simulink model "mainV02_3"  (R2016b)
settings: Solver=VariableStepAuto  StartTime=0.0  StopTime=inf  MaxStep=0.2  RelTol=1e-2
undefined symbols (not defined in the file): checks, delta_e, deltae_degrees, deltat_1, deltat_2, deltat_3, deltat_4, deltat_5, Earth, ft, initialValues, LD, m, Newton, Raphson, s, WGS84
libraries: aerolibutil x8, aerolibasang x5, aerolib6dof2 x4, aerolib6dofsys x3, aerolibtransform2 x3, aerolibbdyn x3, aerolibconvert2 x3, aerolibconvert x2, aerolibatmos2 x1, aerolibobsolete x1, aerolibadyn x1, vrlib x1
(part 2 of 3)

== system mainV02_3/LIBIS Plant/calc alpha_dot ==
  q : Inport
  alpha,beta : Inport  Port=2
  Ab : Inport  Port=3
  Vw : Inport  Port=4
  Constant : Constant  Value=0
  Direction Cosine Matrix Body to Wind : aerolibtransform2/Direction Cosine Matrix Body to Wind
  Product1 : Product  Multiplication=Matrix(*)  SaturateOnIntegerOverflow=on  InputSameDT=on  OutDataTypeStr=Inherit: Same as first input
  Product2 : Product  Inputs=*/  SaturateOnIntegerOverflow=on  InputSameDT=on  OutDataTypeStr=Inherit: Same as first input
  Selector2 : Selector  IndexMode=Zero-based  InputPortWidth=3  IndexOptions=Index vector (dialog)  Indices=2  OutputSizes=1
  Selector3 : Selector  IndexMode=Zero-based  InputPortWidth=3  IndexOptions=Index vector (dialog)  Indices=0  OutputSizes=1
  Sum : Sum  Inputs=++|
  Switch : Switch  Criteria=u2 > Threshold
  Transpose1 : Math  Operator=transpose  SaturateOnIntegerOverflow=on
  Transpose2 : Math  Operator=transpose  SaturateOnIntegerOverflow=on
  alpha_dot : Outport
  wires:
  Direction Cosine Matrix Body to Wind/1 -> Transpose1/1
  Transpose1/1 -> Product1/1
  Product1/1 -> Selector2/1
  Selector2/1 -> Product2/1
  alpha,beta/1 -> Direction Cosine Matrix Body to Wind/1
  q/1 -> Sum/1
  Sum/1 -> alpha_dot/1
  Vw/1 -> Selector3/1
  Selector3/1 -> Switch/2, Product2/2
  Product2/1 -> Switch/1
  Switch/1 -> Sum/2
  Constant/1 -> Switch/3
  Transpose2/1 -> Product1/2
  Ab/1 -> Transpose2/1

== system mainV02_3/Visualization/Airspeed Indicator ==

== system mainV02_3/Visualization/Altimeter ==

== system mainV02_3/Visualization/Artificial Horizon ==

== system mainV02_3/Visualization/Axes to VR Axes ==
  Xe : Inport
  Concatenate : Concatenate  NumInputs=3
  Demux : Demux  Outputs=3
  rad-->deg : Gain  Gain=-1  SaturateOnIntegerOverflow=on  OutDataTypeStr=Inherit: Same as input  ParamDataTypeStr=Inherit: Same as input
  rad-->deg1 : Gain  Gain=-1  SaturateOnIntegerOverflow=on  OutDataTypeStr=Inherit: Same as input  ParamDataTypeStr=Inherit: Same as input
  Xe VR : Outport
  wires:
  Xe/1 -> Demux/1
  Demux/1 -> Concatenate/1
  Demux/2 -> rad-->deg/1
  Demux/3 -> rad-->deg1/1
  Concatenate/1 -> Xe VR/1
  rad-->deg1/1 -> Concatenate/2
  rad-->deg/1 -> Concatenate/3

== system mainV02_3/Visualization/Climb Rate Indicator ==

== system mainV02_3/Visualization/Euler to VR ==
  Euler Angles : Inport
  Axis Angle Vector : Subsystem
  Demux : Demux  Outputs=3
  Mux : Mux  Inputs=2
  Mux1 : Mux  Inputs=2
  Mux2 : Mux  Inputs=2
  Quaternion Multiplication (Pitch & Yaw) : aerolibutil/Quaternion Multiplication
  Quaternion Multiplication (Roll) : aerolibutil/Quaternion Multiplication
  Quaternion Normalization : Subsystem
  Quaternion Normalization1 : Subsystem
  Quaternion Normalization2 : Subsystem
  Vr Pitch Axes : Constant  Value=[0 0 1]
  Vr Roll Axes : Constant  Value=[1 0 0]
  Vr Yaw Axes : Constant  Value=[0 -1 0]
  Axis Angle : Outport
  wires:
  Quaternion Multiplication (Roll)/1 -> Axis Angle Vector/1(e0)
  Quaternion Multiplication (Pitch & Yaw)/1 -> Quaternion Multiplication (Roll)/2
  Axis Angle Vector/1(e0_norm) -> Axis Angle/1
  Quaternion Normalization/1(e0_norm) -> Quaternion Multiplication (Roll)/1
  Quaternion Normalization2/1(e0_norm) -> Quaternion Multiplication (Pitch & Yaw)/1
  Quaternion Normalization1/1(e0_norm) -> Quaternion Multiplication (Pitch & Yaw)/2
  Mux2/1 -> Quaternion Normalization2/1(e0)
  Mux1/1 -> Quaternion Normalization1/1(e0)
  Mux/1 -> Quaternion Normalization/1(e0)
  Demux/3 -> Mux2/1
  Vr Yaw Axes/1 -> Mux2/2
  Demux/2 -> Mux1/1
  Vr Pitch Axes/1 -> Mux1/2
  Demux/1 -> Mux/1
  Vr Roll Axes/1 -> Mux/2
  Euler Angles/1 -> Demux/1

== system mainV02_3/Visualization/Heading Indicator ==

== system mainV02_3/Visualization/Subsystem ==
  "X_ned " : Inport
  Euler_angles : Inport  Port=2
  V_body : Inport  Port=3
  V_ned : Inport  Port=4
  Angle Conversion : aerolibconvert2/Angle Conversion  IU=rad  OU=deg
  Angle Conversion1 : aerolibconvert2/Angle Conversion  IU=rad  OU=deg
  Climbrate : Selector  IndexMode=Zero-based  InputPortWidth=3  IndexOptions=Index vector (dialog)  Indices=2  OutputSizes=1
  Concatenate : Concatenate
  Dot Product : DotProduct  SaturateOnIntegerOverflow=on  OutDataTypeStr=Inherit: Inherit via internal rule
  Flightpath Angle : Subsystem
  Heading : Selector  IndexMode=Zero-based  InputPortWidth=3  IndexOptions=Index vector (dialog)  Indices=2  OutputSizes=1
  Height : Selector  IndexMode=Zero-based  InputPortWidth=3  IndexOptions=Index vector (dialog)  Indices=2  OutputSizes=1
  Length Conversion : aerolibconvert2/Length Conversion  IU=m  OU=ft
  Roll Angle : Selector  IndexMode=Zero-based  InputPortWidth=3  IndexOptions=Index vector (dialog)  Indices=0  OutputSizes=1
  Velocity Conversion : aerolibconvert/Velocity Conversion  IU=m/s  OU=kts
  Velocity Conversion1 : aerolibconvert/Velocity Conversion  IU=m/s  OU=ft/s
  rad-->deg1 : Gain  Gain=-1  SaturateOnIntegerOverflow=on  OutDataTypeStr=Inherit: Same as input  ParamDataTypeStr=Inherit: Same as input
  rad-->deg2 : Gain  Gain=-1  SaturateOnIntegerOverflow=on  OutDataTypeStr=Inherit: Same as input  ParamDataTypeStr=Inherit: Same as input
  rad-->deg3 : Gain  Gain=60  SaturateOnIntegerOverflow=on  OutDataTypeStr=Inherit: Same as input  ParamDataTypeStr=Inherit: Same as input
  vt : Sqrt  SaturateOnIntegerOverflow=on
  Airspeed (kts) : Outport
  Height (ft) : Outport  Port=2
  Roll Flightpath (deg) : Outport  Port=3
  Climb Rate (ft/min) : Outport  Port=4
  Heading (deg) : Outport  Port=5
  wires:
  Velocity Conversion1/1 -> rad-->deg3/1
  rad-->deg3/1 -> Climb Rate (ft/min)/1
  V_ned/1 -> Flightpath Angle/1(Ve), Climbrate/1
  Flightpath Angle/1(gamma) -> Concatenate/2
  rad-->deg2/1 -> Velocity Conversion1/1
  Length Conversion/1 -> Height (ft)/1
  Angle Conversion1/1 -> Roll Flightpath (deg)/1
  Height/1 -> rad-->deg1/1
  Angle Conversion/1 -> Heading (deg)/1  "Heading"
  Heading/1 -> Angle Conversion/1
  Velocity Conversion/1 -> Airspeed (kts)/1
  Dot Product/1 -> vt/1
  Roll Angle/1 -> Concatenate/1
  V_body/1 -> Dot Product/2, Dot Product/1
  Concatenate/1 -> Angle Conversion1/1
  vt/1 -> Velocity Conversion/1
  Climbrate/1 -> rad-->deg2/1
  rad-->deg1/1 -> Length Conversion/1
  Euler_angles/1 -> Roll Angle/1, Heading/1
  "X_ned "/1 -> Height/1

== system mainV02_3/LIBIS Plant/Aerodynamics/CD ==
  prelook-ups : Inport
  plantData : Inport  Port=2
  actuators : Inport  Port=3
  Add : Sum  Inputs=+++++++
  Bus Selector : BusSelector  OutputSignals=alpha,alpha_dot,Omega_body.q
  Bus Selector1 : BusSelector  OutputSignals=alpha,alt,xcg,deltae,deltar,deltafr,deltafl
  Bus Selector2 : BusSelector  OutputSignals=deltae,deltafr,deltafl
  CD0 : Interpolation_n-D  NumberOfTableDimensions=7  Table=LD.Stability.CD0  RequireIndexFractionAsBus=on  InternalRulePriority=Speed
      settings: InputPortMap=u0,u1,u2,u3,u4,u5,u6
  CDalpha : Interpolation_n-D  NumberOfTableDimensions=7  Table=LD.Stability.CDalpha  RequireIndexFractionAsBus=on  InternalRulePriority=Speed
      settings: InputPortMap=u0,u1,u2,u3,u4,u5,u6
  CDalpha_dot : Interpolation_n-D  NumberOfTableDimensions=7  Table=LD.Stability.CDalpha_dot  RequireIndexFractionAsBus=on  InternalRulePriority=Speed
      settings: InputPortMap=u0,u1,u2,u3,u4,u5,u6
  CDdeltae : Interpolation_n-D  NumberOfTableDimensions=7  Table=LD.Stability.CDdeltae  RequireIndexFractionAsBus=on  InternalRulePriority=Speed
      settings: InputPortMap=u0,u1,u2,u3,u4,u5,u6
  CDdeltafl : Interpolation_n-D  NumberOfTableDimensions=7  Table=LD.Stability.CDdeltafl  RequireIndexFractionAsBus=on  InternalRulePriority=Speed
      settings: InputPortMap=u0,u1,u2,u3,u4,u5,u6
  CDdeltafr : Interpolation_n-D  NumberOfTableDimensions=7  Table=LD.Stability.CDdeltafr  RequireIndexFractionAsBus=on  InternalRulePriority=Speed
      settings: InputPortMap=u0,u1,u2,u3,u4,u5,u6
  CDq : Interpolation_n-D  NumberOfTableDimensions=7  Table=LD.Stability.CDq  RequireIndexFractionAsBus=on  InternalRulePriority=Speed
      settings: InputPortMap=u0,u1,u2,u3,u4,u5,u6
  Product{,1..5} (6 alike) : Product
  CD : Outport
  wires:
  prelook-ups/1 -> Bus Selector1/1
  CD0/1 -> Add/1
  Add/1 -> CD/1
  plantData/1 -> Bus Selector/1
  actuators/1 -> Bus Selector2/1
  CDalpha/1 -> Product/1
  Product/1 -> Add/2
  Bus Selector/1 -> Product/2  "<alpha>"
  Bus Selector2/1 -> Product3/2  "<deltae>"
  CDdeltae/1 -> Product3/1
  Product3/1 -> Add/5
  Product2/1 -> Add/4
  Product1/1 -> Add/3
  CDalpha_dot/1 -> Product1/1
  CDq/1 -> Product2/1
  Bus Selector/3 -> Product2/2  "<q>"
  Bus Selector/2 -> Product1/2  "<alpha_dot>"
  Bus Selector1/7 -> CD0/7, CDdeltafl/7, CDdeltafr/7, CDdeltae/7, CDq/7, CDalpha_dot/7, CDalpha/7  "<deltafl>"
  Bus Selector1/6 -> CD0/6, CDdeltafl/6, CDdeltafr/6, CDdeltae/6, CDq/6, CDalpha_dot/6, CDalpha/6  "<deltafr>"
  Bus Selector1/5 -> CD0/5, CDdeltafl/5, CDdeltafr/5, CDdeltae/5, CDq/5, CDalpha_dot/5, CDalpha/5  "<deltar>"
  Bus Selector1/4 -> CD0/4, CDdeltafl/4, CDdeltafr/4, CDdeltae/4, CDq/4, CDalpha_dot/4, CDalpha/4  "<deltae>"
  Bus Selector1/2 -> CD0/2, CDdeltafl/2, CDdeltafr/2, CDdeltae/2, CDq/2, CDalpha_dot/2, CDalpha/2  "<alt>"
  Bus Selector1/3 -> CD0/3, CDdeltafl/3, CDdeltafr/3, CDdeltae/3, CDq/3, CDalpha_dot/3, CDalpha/3  "<xcg>"
  Bus Selector1/1 -> CD0/1, CDdeltafl/1, CDdeltafr/1, CDdeltae/1, CDq/1, CDalpha_dot/1, CDalpha/1  "<alpha>"
  Bus Selector2/3 -> Product5/2  "<deltafl>"
  CDdeltafl/1 -> Product5/1
  Product5/1 -> Add/7
  Product4/1 -> Add/6
  CDdeltafr/1 -> Product4/1
  Bus Selector2/2 -> Product4/2  "<deltafr>"

== system mainV02_3/LIBIS Plant/Aerodynamics/CL ==
  prelook-ups : Inport
  plantData : Inport  Port=2
  actuators1 : Inport  Port=3
  Add : Sum  Inputs=+++++++
  Bus Selector : BusSelector  OutputSignals=alpha,alpha_dot,Omega_body.q
  Bus Selector1 : BusSelector  OutputSignals=alpha,alt,xcg,deltae,deltar,deltafr,deltafl
  Bus Selector3 : BusSelector  OutputSignals=deltae,deltafr,deltafl
  CL0 : Interpolation_n-D  NumberOfTableDimensions=7  Table=LD.Stability.CL0  RequireIndexFractionAsBus=on  InternalRulePriority=Speed
      settings: InputPortMap=u0,u1,u2,u3,u4,u5,u6
  CLalpha : Interpolation_n-D  NumberOfTableDimensions=7  Table=LD.Stability.CLalpha  RequireIndexFractionAsBus=on  InternalRulePriority=Speed
      settings: InputPortMap=u0,u1,u2,u3,u4,u5,u6
  CLalpha_dot : Interpolation_n-D  NumberOfTableDimensions=7  Table=LD.Stability.CLalpha_dot  RequireIndexFractionAsBus=on  InternalRulePriority=Speed
      settings: InputPortMap=u0,u1,u2,u3,u4,u5,u6
  CLdeltae : Interpolation_n-D  NumberOfTableDimensions=7  Table=LD.Stability.CLdeltae  RequireIndexFractionAsBus=on  InternalRulePriority=Speed
      settings: InputPortMap=u0,u1,u2,u3,u4,u5,u6
  CLdeltafl : Interpolation_n-D  NumberOfTableDimensions=7  Table=LD.Stability.CLdeltafl  RequireIndexFractionAsBus=on  InternalRulePriority=Speed
      settings: InputPortMap=u0,u1,u2,u3,u4,u5,u6
  CLdeltafr : Interpolation_n-D  NumberOfTableDimensions=7  Table=LD.Stability.CLdeltafr  RequireIndexFractionAsBus=on  InternalRulePriority=Speed
      settings: InputPortMap=u0,u1,u2,u3,u4,u5,u6
  CLq : Interpolation_n-D  NumberOfTableDimensions=7  Table=LD.Stability.CLq  RequireIndexFractionAsBus=on  InternalRulePriority=Speed
      settings: InputPortMap=u0,u1,u2,u3,u4,u5,u6
  Product{,1..5} (6 alike) : Product
  CL : Outport
  wires:
  prelook-ups/1 -> Bus Selector1/1
  CL0/1 -> Add/1
  Add/1 -> CL/1
  plantData/1 -> Bus Selector/1
  CLalpha/1 -> Product/1
  CLalpha_dot/1 -> Product1/1
  CLq/1 -> Product2/1
  CLdeltae/1 -> Product3/1
  Product/1 -> Add/2
  Product1/1 -> Add/3
  Product2/1 -> Add/4
  Product3/1 -> Add/5
  Bus Selector/1 -> Product/2  "<alpha>"
  Bus Selector/2 -> Product1/2  "<alpha_dot>"
  Bus Selector/3 -> Product2/2  "<q>"
  actuators1/1 -> Bus Selector3/1
  Bus Selector3/3 -> Product5/2  "<deltafl>"
  CLdeltafl/1 -> Product5/1
  Product5/1 -> Add/7
  Product4/1 -> Add/6
  CLdeltafr/1 -> Product4/1
  Bus Selector3/2 -> Product4/2  "<deltafr>"
  Bus Selector3/1 -> Product3/2  "<deltae>"
  Bus Selector1/7 -> CL0/7, CLalpha/7, CLalpha_dot/7, CLdeltafl/7, CLdeltafr/7, CLdeltae/7, CLq/7  "<deltafl>"
  Bus Selector1/6 -> CL0/6, CLalpha/6, CLalpha_dot/6, CLdeltafl/6, CLdeltafr/6, CLdeltae/6, CLq/6  "<deltafr>"
  Bus Selector1/5 -> CL0/5, CLalpha/5, CLalpha_dot/5, CLdeltafl/5, CLdeltafr/5, CLdeltae/5, CLq/5  "<deltar>"
  Bus Selector1/4 -> CL0/4, CLalpha/4, CLalpha_dot/4, CLq/4, CLdeltafl/4, CLdeltafr/4, CLdeltae/4  "<deltae>"
  Bus Selector1/2 -> CL0/2, CLalpha/2, CLalpha_dot/2, CLq/2, CLdeltafl/2, CLdeltafr/2, CLdeltae/2  "<alt>"
  Bus Selector1/3 -> CL0/3, CLalpha/3, CLalpha_dot/3, CLq/3, CLdeltafl/3, CLdeltafr/3, CLdeltae/3  "<xcg>"
  Bus Selector1/1 -> CL0/1, CLalpha/1, CLalpha_dot/1, CLq/1, CLdeltafl/1, CLdeltafr/1, CLdeltae/1  "<alpha>"

== system mainV02_3/LIBIS Plant/Aerodynamics/CY ==
  prelook-ups : Inport
  plantData : Inport  Port=2
  actuators : Inport  Port=3
  Add : Sum  Inputs=++++++
  Bus Selector : BusSelector  OutputSignals=beta,Omega_body.p,Omega_body.r
  Bus Selector1 : BusSelector  OutputSignals=alpha,alt,xcg,deltae,deltar,deltafr,deltafl
  Bus Selector2 : BusSelector  OutputSignals=deltar,deltafr,deltafl
  CYbeta : Interpolation_n-D  NumberOfTableDimensions=7  Table=LD.Stability.CYbeta  RequireIndexFractionAsBus=on  InternalRulePriority=Speed
      settings: InputPortMap=u0,u1,u2,u3,u4,u5,u6
  "CYdeltafl " : Interpolation_n-D  NumberOfTableDimensions=7  Table=LD.Stability.CYdeltafl  RequireIndexFractionAsBus=on  InternalRulePriority=Speed
      settings: InputPortMap=u0,u1,u2,u3,u4,u5,u6
  "CYdeltafr " : Interpolation_n-D  NumberOfTableDimensions=7  Table=LD.Stability.CYdeltafr  RequireIndexFractionAsBus=on  InternalRulePriority=Speed
      settings: InputPortMap=u0,u1,u2,u3,u4,u5,u6
  CYdeltar : Interpolation_n-D  NumberOfTableDimensions=7  Table=LD.Stability.CYdeltar  RequireIndexFractionAsBus=on  InternalRulePriority=Speed
      settings: InputPortMap=u0,u1,u2,u3,u4,u5,u6
  CYp : Interpolation_n-D  NumberOfTableDimensions=7  Table=LD.Stability.CYp  RequireIndexFractionAsBus=on  InternalRulePriority=Speed
      settings: InputPortMap=u0,u1,u2,u3,u4,u5,u6
  CYr : Interpolation_n-D  NumberOfTableDimensions=7  Table=LD.Stability.CYr  RequireIndexFractionAsBus=on  InternalRulePriority=Speed
      settings: InputPortMap=u0,u1,u2,u3,u4,u5,u6
  Product{,1..5} (6 alike) : Product
  CY : Outport
  wires:
  Bus Selector1/7 -> "CYdeltafl "/7, "CYdeltafr "/7, CYdeltar/7, CYr/7, CYp/7, CYbeta/7  "<deltafl>"
  Bus Selector1/6 -> "CYdeltafl "/6, "CYdeltafr "/6, CYdeltar/6, CYr/6, CYp/6, CYbeta/6  "<deltafr>"
  Bus Selector1/5 -> "CYdeltafl "/5, "CYdeltafr "/5, CYdeltar/5, CYr/5, CYp/5, CYbeta/5  "<deltar>"
  prelook-ups/1 -> Bus Selector1/1
  Bus Selector1/4 -> "CYdeltafl "/4, "CYdeltafr "/4, CYdeltar/4, CYr/4, CYp/4, CYbeta/4  "<deltae>"
  Bus Selector1/2 -> "CYdeltafl "/2, "CYdeltafr "/2, CYdeltar/2, CYr/2, CYp/2, CYbeta/2  "<alt>"
  Bus Selector1/3 -> "CYdeltafl "/3, "CYdeltafr "/3, CYdeltar/3, CYr/3, CYp/3, CYbeta/3  "<xcg>"
  Bus Selector1/1 -> "CYdeltafl "/1, "CYdeltafr "/1, CYdeltar/1, CYr/1, CYp/1, CYbeta/1  "<alpha>"
  Add/1 -> CY/1
  plantData/1 -> Bus Selector/1
  actuators/1 -> Bus Selector2/1
  CYbeta/1 -> Product/1
  Product/1 -> Add/1
  Bus Selector/1 -> Product/2  "<beta>"
  Bus Selector2/1 -> Product3/2  "<deltar>"
  CYdeltar/1 -> Product3/1
  Product3/1 -> Add/4
  Product2/1 -> Add/3
  Product1/1 -> Add/2
  CYp/1 -> Product1/1
  CYr/1 -> Product2/1
  Bus Selector/3 -> Product2/2  "<r>"
  Bus Selector/2 -> Product1/2  "<p>"
  "CYdeltafl "/1 -> Product5/1
  Product5/1 -> Add/6
  Product4/1 -> Add/5
  "CYdeltafr "/1 -> Product4/1
  Bus Selector2/2 -> Product4/2  "<deltafr>"
  Bus Selector2/3 -> Product5/2  "<deltafl>"

== system mainV02_3/LIBIS Plant/Aerodynamics/Cl ==
  prelook-ups : Inport
  plantData : Inport  Port=2
  actuators : Inport  Port=3
  Add : Sum  Inputs=++++++
  Bus Selector : BusSelector  OutputSignals=beta,Omega_body.p,Omega_body.r
  Bus Selector1 : BusSelector  OutputSignals=alpha,alt,xcg,deltae,deltar,deltafr,deltafl
  Bus Selector2 : BusSelector  OutputSignals=deltar,deltafr,deltafl
  Clbeta : Interpolation_n-D  NumberOfTableDimensions=7  Table=LD.Stability.Clbeta  RequireIndexFractionAsBus=on  InternalRulePriority=Speed
      settings: InputPortMap=u0,u1,u2,u3,u4,u5,u6
  "Cldeltafl " : Interpolation_n-D  NumberOfTableDimensions=7  Table=LD.Stability.Cldeltafl  RequireIndexFractionAsBus=on  InternalRulePriority=Speed
      settings: InputPortMap=u0,u1,u2,u3,u4,u5,u6
  "Cldeltafr " : Interpolation_n-D  NumberOfTableDimensions=7  Table=LD.Stability.Cldeltafr  RequireIndexFractionAsBus=on  InternalRulePriority=Speed
      settings: InputPortMap=u0,u1,u2,u3,u4,u5,u6
  Cldeltar : Interpolation_n-D  NumberOfTableDimensions=7  Table=LD.Stability.Cldeltar  RequireIndexFractionAsBus=on  InternalRulePriority=Speed
      settings: InputPortMap=u0,u1,u2,u3,u4,u5,u6
  Clp : Interpolation_n-D  NumberOfTableDimensions=7  Table=LD.Stability.Clp  RequireIndexFractionAsBus=on  InternalRulePriority=Speed
      settings: InputPortMap=u0,u1,u2,u3,u4,u5,u6
  Clr : Interpolation_n-D  NumberOfTableDimensions=7  Table=LD.Stability.Clr  RequireIndexFractionAsBus=on  InternalRulePriority=Speed
      settings: InputPortMap=u0,u1,u2,u3,u4,u5,u6
  Product{,1..5} (6 alike) : Product
  Cl : Outport
  wires:
  Bus Selector1/7 -> Clbeta/7, Clp/7, Clr/7, Cldeltar/7, "Cldeltafr "/7, "Cldeltafl "/7  "<deltafl>"
  Bus Selector1/6 -> Clbeta/6, Clp/6, Clr/6, Cldeltar/6, "Cldeltafr "/6, "Cldeltafl "/6  "<deltafr>"
  Bus Selector1/5 -> Clbeta/5, Clp/5, Clr/5, Cldeltar/5, "Cldeltafr "/5, "Cldeltafl "/5  "<deltar>"
  prelook-ups/1 -> Bus Selector1/1
  Bus Selector1/4 -> Clbeta/4, Clp/4, Clr/4, Cldeltar/4, "Cldeltafr "/4, "Cldeltafl "/4  "<deltae>"
  Bus Selector1/2 -> Clbeta/2, Clp/2, Clr/2, Cldeltar/2, "Cldeltafr "/2, "Cldeltafl "/2  "<alt>"
  Bus Selector1/3 -> Clbeta/3, Clp/3, Clr/3, Cldeltar/3, "Cldeltafr "/3, "Cldeltafl "/3  "<xcg>"
  Bus Selector1/1 -> Clbeta/1, Clp/1, Clr/1, Cldeltar/1, "Cldeltafr "/1, "Cldeltafl "/1  "<alpha>"
  Add/1 -> Cl/1
  Clbeta/1 -> Product/1
  Product/1 -> Add/1
  Bus Selector/1 -> Product/2  "<beta>"
  Bus Selector2/1 -> Product3/2  "<deltar>"
  Cldeltar/1 -> Product3/1
  Product3/1 -> Add/4
  Product2/1 -> Add/3
  Product1/1 -> Add/2
  Clp/1 -> Product1/1
  Clr/1 -> Product2/1
  Bus Selector/3 -> Product2/2  "<r>"
  Bus Selector/2 -> Product1/2  "<p>"
  "Cldeltafl "/1 -> Product5/1
  Product5/1 -> Add/6
  Product4/1 -> Add/5
  "Cldeltafr "/1 -> Product4/1
  Bus Selector2/2 -> Product4/2  "<deltafr>"
  Bus Selector2/3 -> Product5/2  "<deltafl>"
  plantData/1 -> Bus Selector/1
  actuators/1 -> Bus Selector2/1

== system mainV02_3/LIBIS Plant/Aerodynamics/Cm ==
  prelook-ups : Inport
  plantData : Inport  Port=2
  actuators1 : Inport  Port=3
  Add1 : Sum  Inputs=+++++++
  Bus Selector : BusSelector  OutputSignals=alpha,alpha_dot,Omega_body.q
  Bus Selector1 : BusSelector  OutputSignals=alpha,alt,xcg,deltae,deltar,deltafr,deltafl
  Bus Selector3 : BusSelector  OutputSignals=deltae,deltafr,deltafl
  Cm0 : Interpolation_n-D  NumberOfTableDimensions=7  Table=LD.Stability.Cm0  RequireIndexFractionAsBus=on  InternalRulePriority=Speed
      settings: InputPortMap=u0,u1,u2,u3,u4,u5,u6
  Cmalpha : Interpolation_n-D  NumberOfTableDimensions=7  Table=LD.Stability.Cmalpha  RequireIndexFractionAsBus=on  InternalRulePriority=Speed
      settings: InputPortMap=u0,u1,u2,u3,u4,u5,u6
  Cmalpha_dot : Interpolation_n-D  NumberOfTableDimensions=7  Table=LD.Stability.Cmalpha_dot  RequireIndexFractionAsBus=on  InternalRulePriority=Speed
      settings: InputPortMap=u0,u1,u2,u3,u4,u5,u6
  Cmdeltae : Interpolation_n-D  NumberOfTableDimensions=7  Table=LD.Stability.Cmdeltae  RequireIndexFractionAsBus=on  InternalRulePriority=Speed
      settings: InputPortMap=u0,u1,u2,u3,u4,u5,u6
  Cmdeltafl : Interpolation_n-D  NumberOfTableDimensions=7  Table=LD.Stability.Cmdeltafl  RequireIndexFractionAsBus=on  InternalRulePriority=Speed
      settings: InputPortMap=u0,u1,u2,u3,u4,u5,u6
  Cmdeltafr : Interpolation_n-D  NumberOfTableDimensions=7  Table=LD.Stability.Cmdeltafr  RequireIndexFractionAsBus=on  InternalRulePriority=Speed
      settings: InputPortMap=u0,u1,u2,u3,u4,u5,u6
  Cmq : Interpolation_n-D  NumberOfTableDimensions=7  Table=LD.Stability.Cmq  RequireIndexFractionAsBus=on  InternalRulePriority=Speed
      settings: InputPortMap=u0,u1,u2,u3,u4,u5,u6
  Product{,1..5} (6 alike) : Product
  Cm : Outport
  wires:
  prelook-ups/1 -> Bus Selector1/1
  Cm0/1 -> Add1/1
  Add1/1 -> Cm/1
  Cmalpha/1 -> Product/1
  Cmalpha_dot/1 -> Product1/1
  Cmq/1 -> Product2/1
  Cmdeltae/1 -> Product3/1
  Product/1 -> Add1/2
  Product1/1 -> Add1/3
  Product2/1 -> Add1/4
  Product3/1 -> Add1/5
  Bus Selector/1 -> Product/2  "<alpha>"
  Bus Selector/2 -> Product1/2  "<alpha_dot>"
  Bus Selector/3 -> Product2/2  "<q>"
  plantData/1 -> Bus Selector/1
  actuators1/1 -> Bus Selector3/1
  Bus Selector3/3 -> Product5/2  "<deltafl>"
  Cmdeltafl/1 -> Product5/1
  Product5/1 -> Add1/7
  Product4/1 -> Add1/6
  Cmdeltafr/1 -> Product4/1
  Bus Selector3/2 -> Product4/2  "<deltafr>"
  Bus Selector3/1 -> Product3/2  "<deltae>"
  Bus Selector1/7 -> Cm0/7, Cmalpha/7, Cmalpha_dot/7, Cmdeltafl/7, Cmdeltafr/7, Cmdeltae/7, Cmq/7  "<deltafl>"
  Bus Selector1/6 -> Cm0/6, Cmalpha/6, Cmalpha_dot/6, Cmdeltafl/6, Cmdeltafr/6, Cmdeltae/6, Cmq/6  "<deltafr>"
  Bus Selector1/5 -> Cm0/5, Cmalpha/5, Cmalpha_dot/5, Cmdeltafl/5, Cmdeltafr/5, Cmdeltae/5, Cmq/5  "<deltar>"
  Bus Selector1/4 -> Cm0/4, Cmalpha/4, Cmalpha_dot/4, Cmdeltafl/4, Cmdeltafr/4, Cmdeltae/4, Cmq/4  "<deltae>"
  Bus Selector1/2 -> Cm0/2, Cmalpha/2, Cmalpha_dot/2, Cmq/2, Cmdeltafl/2, Cmdeltafr/2, Cmdeltae/2  "<alt>"
  Bus Selector1/3 -> Cm0/3, Cmalpha/3, Cmalpha_dot/3, Cmdeltafl/3, Cmdeltafr/3, Cmdeltae/3, Cmq/3  "<xcg>"
  Bus Selector1/1 -> Cm0/1, Cmalpha/1, Cmalpha_dot/1, Cmq/1, Cmdeltafl/1, Cmdeltafr/1, Cmdeltae/1  "<alpha>"

== system mainV02_3/LIBIS Plant/Aerodynamics/Cn ==
  prelook-ups : Inport
  plantData : Inport  Port=2
  actuators : Inport  Port=3
  Add : Sum  Inputs=++++++
  Bus Selector : BusSelector  OutputSignals=beta,Omega_body.p,Omega_body.r
  Bus Selector1 : BusSelector  OutputSignals=alpha,alt,xcg,deltae,deltar,deltafr,deltafl
  Bus Selector2 : BusSelector  OutputSignals=deltar,deltafr,deltafl
  Cnbeta : Interpolation_n-D  NumberOfTableDimensions=7  Table=LD.Stability.Cnbeta  RequireIndexFractionAsBus=on  InternalRulePriority=Speed
      settings: InputPortMap=u0,u1,u2,u3,u4,u5,u6
  "Cndeltafl " : Interpolation_n-D  NumberOfTableDimensions=7  Table=LD.Stability.Cndeltafl  RequireIndexFractionAsBus=on  InternalRulePriority=Speed
      settings: InputPortMap=u0,u1,u2,u3,u4,u5,u6
  "Cndeltafr " : Interpolation_n-D  NumberOfTableDimensions=7  Table=LD.Stability.Cndeltafr  RequireIndexFractionAsBus=on  InternalRulePriority=Speed
      settings: InputPortMap=u0,u1,u2,u3,u4,u5,u6
  Cndeltar : Interpolation_n-D  NumberOfTableDimensions=7  Table=LD.Stability.Cndeltar  RequireIndexFractionAsBus=on  InternalRulePriority=Speed
      settings: InputPortMap=u0,u1,u2,u3,u4,u5,u6
  Cnp : Interpolation_n-D  NumberOfTableDimensions=7  Table=LD.Stability.Cnp  RequireIndexFractionAsBus=on  InternalRulePriority=Speed
      settings: InputPortMap=u0,u1,u2,u3,u4,u5,u6
  Cnr : Interpolation_n-D  NumberOfTableDimensions=7  Table=LD.Stability.Cnr  RequireIndexFractionAsBus=on  InternalRulePriority=Speed
      settings: InputPortMap=u0,u1,u2,u3,u4,u5,u6
  Product{,1..5} (6 alike) : Product
  Cn : Outport
  wires:
  Bus Selector1/7 -> Cnp/7, Cnr/7, Cndeltar/7, "Cndeltafr "/7, "Cndeltafl "/7, Cnbeta/7  "<deltafl>"
  Bus Selector1/6 -> Cnp/6, Cnr/6, Cndeltar/6, "Cndeltafr "/6, "Cndeltafl "/6, Cnbeta/6  "<deltafr>"
  Bus Selector1/5 -> Cnp/5, Cnr/5, Cndeltar/5, "Cndeltafr "/5, "Cndeltafl "/5, Cnbeta/5  "<deltar>"
  prelook-ups/1 -> Bus Selector1/1
  Bus Selector1/4 -> Cnp/4, Cnr/4, Cndeltar/4, "Cndeltafr "/4, "Cndeltafl "/4, Cnbeta/4  "<deltae>"
  Bus Selector1/2 -> Cnp/2, Cnr/2, Cndeltar/2, "Cndeltafr "/2, "Cndeltafl "/2, Cnbeta/2  "<alt>"
  Bus Selector1/3 -> Cnp/3, Cnr/3, Cndeltar/3, "Cndeltafr "/3, "Cndeltafl "/3, Cnbeta/3  "<xcg>"
  Bus Selector1/1 -> Cnp/1, Cnr/1, Cndeltar/1, "Cndeltafr "/1, "Cndeltafl "/1, Cnbeta/1  "<alpha>"
  Add/1 -> Cn/1
  plantData/1 -> Bus Selector/1
  actuators/1 -> Bus Selector2/1
  Cnbeta/1 -> Product/1
  Product/1 -> Add/1
  Bus Selector/1 -> Product/2  "<beta>"
  Bus Selector2/1 -> Product3/2  "<deltar>"
  Cndeltar/1 -> Product3/1
  Product3/1 -> Add/4
  Product2/1 -> Add/3
  Product1/1 -> Add/2
  Cnp/1 -> Product1/1
  Cnr/1 -> Product2/1
  Bus Selector/3 -> Product2/2  "<r>"
  Bus Selector/2 -> Product1/2  "<p>"
  "Cndeltafl "/1 -> Product5/1
  Product5/1 -> Add/6
  Product4/1 -> Add/5
  "Cndeltafr "/1 -> Product4/1
  Bus Selector2/2 -> Product4/2  "<deltafr>"
  Bus Selector2/3 -> Product5/2  "<deltafl>"

== system mainV02_3/LIBIS Plant/Aerodynamics/DerivedConditions ==
  Speed of Sound : Inport
  Air Density : Inport  Port=2
  WindVelocity : Inport  Port=3  PortDimensions=3
  WindAngularRates : Inport  Port=4  PortDimensions=3
  Vb : Inport  Port=5  PortDimensions=3
  Dynamic Pressure : aerolibasang/Dynamic Pressure
  Mach Number : aerolibasang/Mach Number
  Sum2 : Sum  Inputs=|+-  SaturateOnIntegerOverflow=on  InputSameDT=on  OutDataTypeStr=Inherit: Same as first input
  Mach : Outport
  qbar : Outport  Port=2  InitialOutput=0
  "pqrWind " : Outport  Port=3
  wires:
  Speed of Sound/1 -> Mach Number/2  "speedSound"
  Mach Number/1 -> Mach/1  "Mach"
  Air Density/1 -> Dynamic Pressure/2
  Dynamic Pressure/1 -> qbar/1  "qbar"
  WindAngularRates/1 -> "pqrWind "/1
  Vb/1 -> Sum2/1  "V_body"
  Sum2/1 -> Dynamic Pressure/1, Mach Number/1  "V_ground"
  WindVelocity/1 -> Sum2/2  "V_wind"

== system mainV02_3/LIBIS Plant/Propulsion/8S 25C Battery ==
  note: ZIPPY Compact 5800mAh 8S 25C Lipo Pack
      |
      | Spec.
      | Capacity: 5800mAh
      | Voltage: 8S1P / 8 Cell / 29.6V
      | Discharge: 25C Constant / 35C Burst
      | Weight: 1025g (including wire, plug & case)
      | Dimensions: 167x46x64mm
      | Balance Plug: JST-XH
      | Discharge Plug: 5.5mm Bullet
  note: ZIPPY Compact 5800mAh 8S 25C Lipo Pack
      |
      | SKU
      | ZC.5800.8S.25
      | Weight(g):
      | 1020.00
      | Length:
      | 161.00
      | Width
      | 46.00
      | Height
      | 73.00
      | Capacity (mAh):
      | 5800.00
      | Discharge(c):
      | 25.00
      | Length-A(mm)
      | 167.00
      | Height-B(mm)
      | 46.00
      | Width-C(mm):
      | 64.00
      | Unit Weight (g):
      | 1020
      | Max Charge Rate(C)
      | 5.00
      | Watt Hour
      | 171.00
  note: Batería escogida: 8S 29.6V
  Battery_Capacity : Constant  Value=5.8
  Battery_Voltage : Constant  Value=29.6
  Max_discharge_rate : Constant  Value=145
  profundidad_descarga : Constant  Value=0.95
  rendimiento_bateria : Constant  Value=0.98
  C_battery : Outport  Unit=A*h
  deep_discharge_battery : Outport  Port=2  Unit=1
  V_battery : Outport  Port=3  Unit=V
  eta_battery : Outport  Port=4  Unit=1
  max_discharge_rate : Outport  Port=5  Unit=A*h
  wires:
  Battery_Voltage/1 -> V_battery/1
  Battery_Capacity/1 -> C_battery/1
  profundidad_descarga/1 -> deep_discharge_battery/1
  rendimiento_bateria/1 -> eta_battery/1
  Max_discharge_rate/1 -> max_discharge_rate/1

== system mainV02_3/LIBIS Plant/Propulsion/Motor_1 ==
  Vbattery : Inport
  Throttle : Inport  Port=2
  plantData : Inport  Port=3
  3x3 Cross Product : aerolibutil/3x3 Cross Product
  Bus Selector : BusSelector  OutputSignals=V_body,CG,LLA.Altitude_m
  Constant1 : Constant  Value=0
  Constant2 : Constant  Value=0
  ESC_1 : Subsystem
  Motor and Propeller Coupling_1 : Subsystem
  Mux : Mux  Inputs=3
  Selector2 : Selector  InputPortWidth=3  IndexOptions=Index vector (dialog)  Indices=[1]  OutputSizes=1
  Sum1 : Sum  Inputs=+-|
  Terminator : Terminator
  Terminator1 : Terminator
  "motor2 position " : Constant  Value=LD.Propulsion.motor1.Position
  Im : Outport
  Thrust : Outport  Port=2
  Thrust_moment : Outport  Port=3
  wires:
  Throttle/1 -> ESC_1/2(Throttle)
  Vbattery/1 -> ESC_1/1(V_battery)
  ESC_1/1(V_ESC) -> Motor and Propeller Coupling_1/1(Voltage)  "V_ESC"
  Selector2/1 -> Motor and Propeller Coupling_1/3(Vflight)
  [V_body] -> Selector2/1
  Sum1/1 -> 3x3 Cross Product/1  "arm"
  Mux/1 -> Thrust/1, 3x3 Cross Product/2  "Thrust_vector"
  Constant1/1 -> Mux/2
  3x3 Cross Product/1 -> Thrust_moment/1
  plantData/1 -> Bus Selector/1
  Bus Selector/1 -> [V_body]  "<V_body>"
  Bus Selector/2 -> [CG]  "<CG>"
  Motor and Propeller Coupling_1/1(Thrust) -> Mux/1  "Thrust_scalar"
  Bus Selector/3 -> [Altitude]  "<Altitude_m>"
  [CG] -> Sum1/2
  "motor2 position "/1 -> Sum1/1
  Motor and Propeller Coupling_1/3(Current) -> Im/1
  [Altitude] -> Motor and Propeller Coupling_1/2(Height)
  Motor and Propeller Coupling_1/2(Power) -> Terminator/1
  Motor and Propeller Coupling_1/4(RPM) -> Terminator1/1
  Constant2/1 -> Mux/3

== system mainV02_3/LIBIS Plant/Propulsion/Motor_2 ==
  Vbattery : Inport
  Throttle : Inport  Port=2
  plantData : Inport  Port=3
  3x3 Cross Product : aerolibutil/3x3 Cross Product
  Bus Selector : BusSelector  OutputSignals=V_body,CG,LLA.Altitude_m
  Constant1 : Constant  Value=0
  Constant2 : Constant  Value=0
  ESC_2 : Subsystem
  Motor and Propeller Coupling_2 : Subsystem
  Mux : Mux  Inputs=3
  Selector2 : Selector  InputPortWidth=3  IndexOptions=Index vector (dialog)  Indices=[3]  OutputSizes=1
  Sum1 : Sum  Inputs=+-|
  Terminator : Terminator
  Terminator1 : Terminator
  Unary Minus : UnaryMinus
  "motor2 position " : Constant  Value=LD.Propulsion.motor2.Position
  Im : Outport
  Thrust : Outport  Port=2
  Thrust_moment : Outport  Port=3
  wires:
  Throttle/1 -> ESC_2/2(Throttle)
  Vbattery/1 -> ESC_2/1(V_battery)
  ESC_2/1(V_ESC) -> Motor and Propeller Coupling_2/1(Voltage)  "V_ESC"
  Selector2/1 -> Motor and Propeller Coupling_2/3(Vflight)
  [V_body] -> Selector2/1
  Sum1/1 -> 3x3 Cross Product/1  "arm"
  Mux/1 -> Thrust/1, 3x3 Cross Product/2  "Thrust_vector"
  Constant1/1 -> Mux/2
  3x3 Cross Product/1 -> Thrust_moment/1
  Constant2/1 -> Mux/1
  plantData/1 -> Bus Selector/1
  Bus Selector/1 -> [V_body]  "<V_body>"
  Bus Selector/2 -> [CG]  "<CG>"
  Motor and Propeller Coupling_2/1(Thrust) -> Unary Minus/1  "Thrust_scalar"
  Unary Minus/1 -> Mux/3
  Bus Selector/3 -> [Altitude]  "<Altitude_m>"
  [CG] -> Sum1/2
  "motor2 position "/1 -> Sum1/1
  Motor and Propeller Coupling_2/3(Current) -> Im/1
  [Altitude] -> Motor and Propeller Coupling_2/2(Height)
  Motor and Propeller Coupling_2/2(Power) -> Terminator/1
  Motor and Propeller Coupling_2/4(RPM) -> Terminator1/1

== system mainV02_3/LIBIS Plant/Propulsion/Motor_3 ==
  Vbattery : Inport
  Throttle : Inport  Port=2
  plantData : Inport  Port=3
  3x3 Cross Product : aerolibutil/3x3 Cross Product
  Bus Selector : BusSelector  OutputSignals=V_body,CG,LLA.Altitude_m
  Constant1 : Constant  Value=0
  Constant2 : Constant  Value=0
  ESC_3 : Subsystem
  Motor and Propeller Coupling_3 : Subsystem
  Mux : Mux  Inputs=3
  Selector2 : Selector  InputPortWidth=3  IndexOptions=Index vector (dialog)  Indices=[3]  OutputSizes=1
  Sum1 : Sum  Inputs=+-|
  Terminator : Terminator
  Terminator1 : Terminator
  Unary Minus : UnaryMinus
  "motor2 position " : Constant  Value=LD.Propulsion.motor3.Position
  Im : Outport
  Thrust : Outport  Port=2
  Thrust_moment : Outport  Port=3
  wires:
  Throttle/1 -> ESC_3/2(Throttle)
  Vbattery/1 -> ESC_3/1(V_battery)
  ESC_3/1(V_ESC) -> Motor and Propeller Coupling_3/1(Voltage)  "V_ESC"
  Selector2/1 -> Motor and Propeller Coupling_3/3(Vflight)
  [V_body] -> Selector2/1
  Sum1/1 -> 3x3 Cross Product/1  "arm"
  Mux/1 -> Thrust/1, 3x3 Cross Product/2  "Thrust_vector"
  Constant1/1 -> Mux/2
  3x3 Cross Product/1 -> Thrust_moment/1
  Constant2/1 -> Mux/1
  plantData/1 -> Bus Selector/1
  Bus Selector/1 -> [V_body]  "<V_body>"
  Bus Selector/2 -> [CG]  "<CG>"
  Motor and Propeller Coupling_3/1(Thrust) -> Unary Minus/1  "Thrust_scalar"
  Unary Minus/1 -> Mux/3
  Bus Selector/3 -> [Altitude]  "<Altitude_m>"
  [CG] -> Sum1/2
  "motor2 position "/1 -> Sum1/1
  Motor and Propeller Coupling_3/3(Current) -> Im/1
  [Altitude] -> Motor and Propeller Coupling_3/2(Height)
  Motor and Propeller Coupling_3/2(Power) -> Terminator/1
  Motor and Propeller Coupling_3/4(RPM) -> Terminator1/1

== system mainV02_3/LIBIS Plant/Propulsion/Motor_4 ==
  Vbattery : Inport
  Throttle : Inport  Port=2
  plantData : Inport  Port=3
  3x3 Cross Product : aerolibutil/3x3 Cross Product
  Bus Selector : BusSelector  OutputSignals=V_body,CG,LLA.Altitude_m
  Constant1 : Constant  Value=0
  Constant2 : Constant  Value=0
  ESC_4 : Subsystem
  Motor and Propeller Coupling_4 : Subsystem
  Mux : Mux  Inputs=3
  Selector2 : Selector  InputPortWidth=3  IndexOptions=Index vector (dialog)  Indices=[3]  OutputSizes=1
  Sum1 : Sum  Inputs=+-|
  Terminator : Terminator
  Terminator1 : Terminator
  Unary Minus : UnaryMinus
  "motor2 position " : Constant  Value=LD.Propulsion.motor4.Position
  Im : Outport
  Thrust : Outport  Port=2
  Thrust_moment : Outport  Port=3
  wires:
  Throttle/1 -> ESC_4/2(Throttle)
  Vbattery/1 -> ESC_4/1(V_battery)
  ESC_4/1(V_ESC) -> Motor and Propeller Coupling_4/1(Voltage)  "V_ESC"
  Selector2/1 -> Motor and Propeller Coupling_4/3(Vflight)
  [V_body] -> Selector2/1
  Sum1/1 -> 3x3 Cross Product/1  "arm"
  Mux/1 -> Thrust/1, 3x3 Cross Product/2  "Thrust_vector"
  Constant1/1 -> Mux/2
  3x3 Cross Product/1 -> Thrust_moment/1
  Constant2/1 -> Mux/1
  plantData/1 -> Bus Selector/1
  Bus Selector/1 -> [V_body]  "<V_body>"
  Bus Selector/2 -> [CG]  "<CG>"
  Motor and Propeller Coupling_4/1(Thrust) -> Unary Minus/1  "Thrust_scalar"
  Unary Minus/1 -> Mux/3
  Bus Selector/3 -> [Altitude]  "<Altitude_m>"
  [CG] -> Sum1/2
  "motor2 position "/1 -> Sum1/1
  Motor and Propeller Coupling_4/3(Current) -> Im/1
  [Altitude] -> Motor and Propeller Coupling_4/2(Height)
  Motor and Propeller Coupling_4/2(Power) -> Terminator/1
  Motor and Propeller Coupling_4/4(RPM) -> Terminator1/1

== system mainV02_3/LIBIS Plant/Propulsion/Motor_5 ==
  Vbattery : Inport
  Throttle : Inport  Port=2
  plantData : Inport  Port=3
  3x3 Cross Product : aerolibutil/3x3 Cross Product
  Bus Selector : BusSelector  OutputSignals=V_body,CG,LLA.Altitude_m
  Constant1 : Constant  Value=0
  Constant2 : Constant  Value=0
  ESC_5 : Subsystem
  Motor and Propeller Coupling_5 : Subsystem
  Mux : Mux  Inputs=3
  Selector2 : Selector  InputPortWidth=3  IndexOptions=Index vector (dialog)  Indices=[3]  OutputSizes=1
  Sum1 : Sum  Inputs=+-|
  Terminator : Terminator
  Terminator1 : Terminator
  Unary Minus : UnaryMinus
  "motor2 position " : Constant  Value=LD.Propulsion.motor5.Position
  Im : Outport
  Thrust : Outport  Port=2
  Thrust_moment : Outport  Port=3
  wires:
  Throttle/1 -> ESC_5/2(Throttle)
  Vbattery/1 -> ESC_5/1(V_battery)
  ESC_5/1(V_ESC) -> Motor and Propeller Coupling_5/1(Voltage)  "V_ESC"
  Selector2/1 -> Motor and Propeller Coupling_5/3(Vflight)
  [V_body] -> Selector2/1
  Sum1/1 -> 3x3 Cross Product/1  "arm"
  Mux/1 -> Thrust/1, 3x3 Cross Product/2  "Thrust_vector"
  Constant1/1 -> Mux/2
  3x3 Cross Product/1 -> Thrust_moment/1
  Constant2/1 -> Mux/1
  plantData/1 -> Bus Selector/1
  Bus Selector/1 -> [V_body]  "<V_body>"
  Bus Selector/2 -> [CG]  "<CG>"
  Motor and Propeller Coupling_5/1(Thrust) -> Unary Minus/1  "Thrust_scalar"
  Unary Minus/1 -> Mux/3
  Bus Selector/3 -> [Altitude]  "<Altitude_m>"
  [CG] -> Sum1/2
  "motor2 position "/1 -> Sum1/1
  Motor and Propeller Coupling_5/3(Current) -> Im/1
  [Altitude] -> Motor and Propeller Coupling_5/2(Height)
  Motor and Propeller Coupling_5/2(Power) -> Terminator/1
  Motor and Propeller Coupling_5/4(RPM) -> Terminator1/1

== system mainV02_3/Visualization/Euler to VR/Axis Angle Vector ==
  e0 : Inport
  2 : Gain  Gain=2  SaturateOnIntegerOverflow=on  OutDataTypeStr=Inherit: Same as input  ParamDataTypeStr=Inherit: Same as input
  Concatenate : Concatenate
  Demux : Demux  Outputs=[1 3 ]
  Product : Product  Inputs=*/  SaturateOnIntegerOverflow=on  InputSameDT=on  OutDataTypeStr=Inherit: Same as first input
  Trigonometric Function : Trigonometry
  Trigonometric Function2 : Trigonometry  Operator=acos
  e0_norm : Outport
  wires:
  Demux/1 -> Trigonometric Function2/1
  Demux/2 -> Product/1
  Concatenate/1 -> e0_norm/1
  Product/1 -> Concatenate/1
  2/1 -> Concatenate/2
  Trigonometric Function/1 -> Product/2
  Trigonometric Function2/1 -> Trigonometric Function/1, 2/1
  e0/1 -> Demux/1

== system mainV02_3/Visualization/Euler to VR/Quaternion Normalization ==
  e0 : Inport
  1/2 : Gain  Gain=1/2  SaturateOnIntegerOverflow=on  OutDataTypeStr=Inherit: Same as input  ParamDataTypeStr=Inherit: Same as input
  Concatenate : Concatenate
  Demux : Demux  Outputs=[1 3]
  Product : Product  SaturateOnIntegerOverflow=on  InputSameDT=on  OutDataTypeStr=Inherit: Same as first input
  Trigonometric Function : Trigonometry
  Trigonometric Function1 : Trigonometry  Operator=cos
  e0_norm : Outport
  wires:
  Trigonometric Function1/1 -> Concatenate/1
  Demux/2 -> Product/2
  Demux/1 -> 1/2/1
  Concatenate/1 -> e0_norm/1
  Product/1 -> Concatenate/2
  Trigonometric Function/1 -> Product/1
  1/2/1 -> Trigonometric Function1/1, Trigonometric Function/1
  e0/1 -> Demux/1

== system mainV02_3/Visualization/Euler to VR/Quaternion Normalization1 ==
  e0 : Inport
  1/2 : Gain  Gain=1/2  SaturateOnIntegerOverflow=on  OutDataTypeStr=Inherit: Same as input  ParamDataTypeStr=Inherit: Same as input
  Concatenate : Concatenate
  Demux : Demux  Outputs=[1 3]
  Product : Product  SaturateOnIntegerOverflow=on  InputSameDT=on  OutDataTypeStr=Inherit: Same as first input
  Trigonometric Function : Trigonometry
  Trigonometric Function1 : Trigonometry  Operator=cos
  e0_norm : Outport
  wires:
  e0/1 -> Demux/1
  1/2/1 -> Trigonometric Function/1, Trigonometric Function1/1
  Trigonometric Function/1 -> Product/1
  Product/1 -> Concatenate/2
  Concatenate/1 -> e0_norm/1
  Demux/1 -> 1/2/1
  Demux/2 -> Product/2
  Trigonometric Function1/1 -> Concatenate/1

== system mainV02_3/Visualization/Euler to VR/Quaternion Normalization2 ==
  e0 : Inport
  1/2 : Gain  Gain=1/2  SaturateOnIntegerOverflow=on  OutDataTypeStr=Inherit: Same as input  ParamDataTypeStr=Inherit: Same as input
  Concatenate : Concatenate
  Demux : Demux  Outputs=[1 3]
  Product : Product  SaturateOnIntegerOverflow=on  InputSameDT=on  OutDataTypeStr=Inherit: Same as first input
  Trigonometric Function : Trigonometry
  Trigonometric Function1 : Trigonometry  Operator=cos
  e0_norm : Outport
  wires:
  Trigonometric Function1/1 -> Concatenate/1
  Demux/2 -> Product/2
  Demux/1 -> 1/2/1
  Concatenate/1 -> e0_norm/1
  Product/1 -> Concatenate/2
  Trigonometric Function/1 -> Product/1
  1/2/1 -> Trigonometric Function1/1, Trigonometric Function/1
  e0/1 -> Demux/1

== system mainV02_3/Visualization/Subsystem/Flightpath Angle ==
  Ve : Inport
  Constant : Constant  Value=0
  Sum2 : Sum  Inputs=+  SaturateOnIntegerOverflow=on  InputSameDT=on  OutDataTypeStr=Inherit: Same as first input
  Switch : Switch  Criteria=u2 > Threshold
  product : Product  SaturateOnIntegerOverflow=on  InputSameDT=on  OutDataTypeStr=Inherit: Same as first input
  product1 : Product  Inputs=/*  SaturateOnIntegerOverflow=on  InputSameDT=on  OutDataTypeStr=Inherit: Same as first input
  rad-->deg4 : Gain  Gain=-1  SaturateOnIntegerOverflow=on  OutDataTypeStr=Inherit: Same as input  ParamDataTypeStr=Inherit: Same as input
  tangent : Trigonometry  Operator=atan
  u,v : Selector  IndexMode=Zero-based  InputPortWidth=3  IndexOptions=Index vector (dialog)  Indices=[0 1]  OutputSizes=1
  v : Sqrt  SaturateOnIntegerOverflow=on
  w : Selector  IndexMode=Zero-based  InputPortWidth=3  IndexOptions=Index vector (dialog)  Indices=2  OutputSizes=1
  gamma : Outport
  wires:
  Ve/1 -> w/1, u,v/1
  product/1 -> Sum2/1
  Sum2/1 -> v/1
  product1/1 -> tangent/1
  u,v/1 -> product/2, product/1
  w/1 -> rad-->deg4/1
  v/1 -> Switch/2, product1/1
  rad-->deg4/1 -> product1/2
  tangent/1 -> Switch/1
  Constant/1 -> Switch/3
  Switch/1 -> gamma/1

== system mainV02_3/LIBIS Plant/Propulsion/Motor_1/ESC_1 ==
  V_battery : Inport  Unit=V
  Throttle : Inport  Port=2  Unit=1
  Product : Product
  Product1 : Product
  eta_ESC : Constant  Value=LD.Propulsion.ESC1.eta
  isActive : Subsystem  Commented=on
  V_ESC : Outport  Unit=V
  wires:
  eta_ESC/1 -> Product/2
  V_battery/1 -> Product/1
  Product/1 -> Product1/1
  Product1/1 -> V_ESC/1
  Throttle/1 -> Product1/2

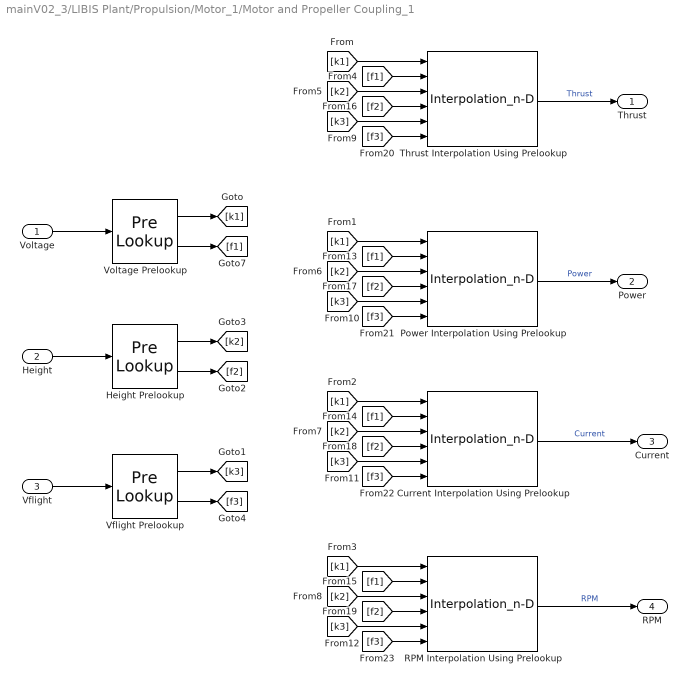
== system mainV02_3/LIBIS Plant/Propulsion/Motor_1/Motor and Propeller Coupling_1 ==
  Voltage : Inport
  Height : Inport  Port=2
  Vflight : Inport  Port=3
  Current Interpolation Using Prelookup : Interpolation_n-D  NumberOfTableDimensions=3  Table=LD.Propulsion.motor1.Current  DiagnosticForOutOfRangeInput=Warning  InternalRulePriority=Speed
      settings: InputPortMap=u0,u1,u2,u3,u4,u5
  Height Prelookup : PreLookup  BreakpointsData=LD.Propulsion.motor1.Height  ExtrapMethod=Linear  DiagnosticForOutOfRangeInput=Warning
  Power Interpolation Using Prelookup : Interpolation_n-D  NumberOfTableDimensions=3  Table=LD.Propulsion.motor1.Power  DiagnosticForOutOfRangeInput=Warning  InternalRulePriority=Speed
      settings: InputPortMap=u0,u1,u2,u3,u4,u5
  RPM Interpolation Using Prelookup : Interpolation_n-D  NumberOfTableDimensions=3  Table=LD.Propulsion.motor1.RPM  DiagnosticForOutOfRangeInput=Warning  InternalRulePriority=Speed
      settings: InputPortMap=u0,u1,u2,u3,u4,u5
  Thrust Interpolation Using Prelookup : Interpolation_n-D  NumberOfTableDimensions=3  Table=LD.Propulsion.motor1.Thrust  DiagnosticForOutOfRangeInput=Warning  InternalRulePriority=Speed
      settings: InputPortMap=u0,u1,u2,u3,u4,u5
  Vflight Prelookup : PreLookup  BreakpointsData=LD.Propulsion.motor1.Vflight  ExtrapMethod=Linear  DiagnosticForOutOfRangeInput=Warning
  Voltage Prelookup : PreLookup  BreakpointsData=LD.Propulsion.motor1.Voltage  ExtrapMethod=Linear  DiagnosticForOutOfRangeInput=Warning
  Thrust : Outport
  Power : Outport  Port=2
  Current : Outport  Port=3
  RPM : Outport  Port=4
  wires:
  Height/1 -> Height Prelookup/1
  Vflight/1 -> Vflight Prelookup/1
  RPM Interpolation Using Prelookup/1 -> RPM/1  "RPM"
  Power Interpolation Using Prelookup/1 -> Power/1  "Power"
  Thrust Interpolation Using Prelookup/1 -> Thrust/1  "Thrust"
  Current Interpolation Using Prelookup/1 -> Current/1  "Current"
  Voltage/1 -> Voltage Prelookup/1
  Voltage Prelookup/1 -> [k1]
  Voltage Prelookup/2 -> [f1]
  Height Prelookup/1 -> [k2]
  Height Prelookup/2 -> [f2]
  Vflight Prelookup/2 -> [f3]
  Vflight Prelookup/1 -> [k3]
  [k1] -> Thrust Interpolation Using Prelookup/1
  [k1] -> Power Interpolation Using Prelookup/1
  [k1] -> Current Interpolation Using Prelookup/1
  [k1] -> RPM Interpolation Using Prelookup/1
  [f1] -> Thrust Interpolation Using Prelookup/2
  [k2] -> Thrust Interpolation Using Prelookup/3
  [k2] -> Power Interpolation Using Prelookup/3
  [k2] -> Current Interpolation Using Prelookup/3
  [k2] -> RPM Interpolation Using Prelookup/3
  [k3] -> Thrust Interpolation Using Prelookup/5
  [k3] -> Power Interpolation Using Prelookup/5
  [k3] -> Current Interpolation Using Prelookup/5
  [k3] -> RPM Interpolation Using Prelookup/5
  [f1] -> Power Interpolation Using Prelookup/2
  [f1] -> Current Interpolation Using Prelookup/2
  [f1] -> RPM Interpolation Using Prelookup/2
  [f2] -> RPM Interpolation Using Prelookup/4
  [f2] -> Current Interpolation Using Prelookup/4
  [f2] -> Power Interpolation Using Prelookup/4
  [f2] -> Thrust Interpolation Using Prelookup/4
  [f3] -> RPM Interpolation Using Prelookup/6
  [f3] -> Current Interpolation Using Prelookup/6
  [f3] -> Power Interpolation Using Prelookup/6
  [f3] -> Thrust Interpolation Using Prelookup/6

== system mainV02_3/LIBIS Plant/Propulsion/Motor_2/ESC_2 ==
  V_battery : Inport  Unit=V
  Throttle : Inport  Port=2  Unit=1
  Product : Product
  Product1 : Product
  eta_ESC : Constant  Value=LD.Propulsion.ESC2.eta
  isActive : Subsystem  Commented=on
  V_ESC : Outport  Unit=V
  wires:
  eta_ESC/1 -> Product/2
  V_battery/1 -> Product/1
  Product/1 -> Product1/1
  Product1/1 -> V_ESC/1
  Throttle/1 -> Product1/2

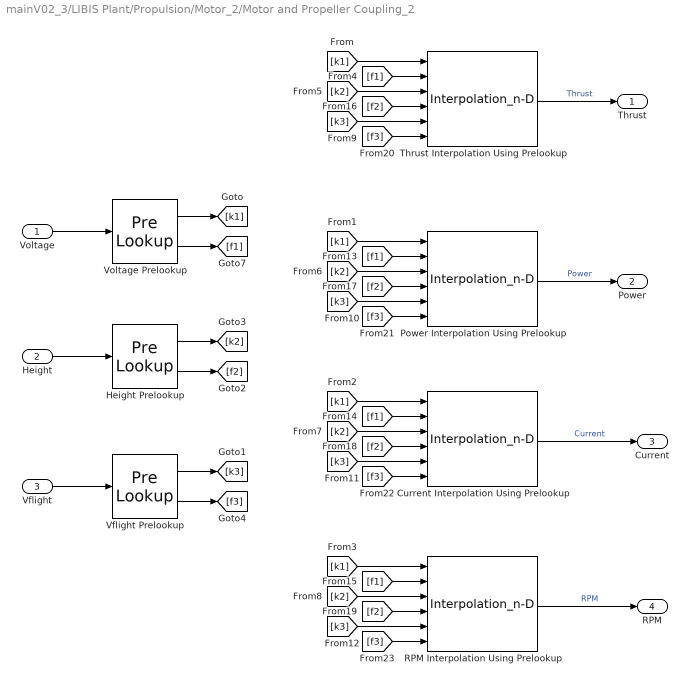
== system mainV02_3/LIBIS Plant/Propulsion/Motor_2/Motor and Propeller Coupling_2 ==
  Voltage : Inport
  Height : Inport  Port=2
  Vflight : Inport  Port=3
  Current Interpolation Using Prelookup : Interpolation_n-D  NumberOfTableDimensions=3  Table=LD.Propulsion.motor2.Current  ExtrapMethod=Clip  DiagnosticForOutOfRangeInput=Warning  InternalRulePriority=Speed
      settings: InputPortMap=u0,u1,u2,u3,u4,u5
  Height Prelookup : PreLookup  BreakpointsData=LD.Propulsion.motor2.Height  ExtrapMethod=Linear
  Power Interpolation Using Prelookup : Interpolation_n-D  NumberOfTableDimensions=3  Table=LD.Propulsion.motor2.Power  ExtrapMethod=Clip  DiagnosticForOutOfRangeInput=Warning  InternalRulePriority=Speed
      settings: InputPortMap=u0,u1,u2,u3,u4,u5
  RPM Interpolation Using Prelookup : Interpolation_n-D  NumberOfTableDimensions=3  Table=LD.Propulsion.motor2.RPM  ExtrapMethod=Clip  DiagnosticForOutOfRangeInput=Warning  InternalRulePriority=Speed
      settings: InputPortMap=u0,u1,u2,u3,u4,u5
  Thrust Interpolation Using Prelookup : Interpolation_n-D  NumberOfTableDimensions=3  Table=LD.Propulsion.motor2.Thrust  ExtrapMethod=Clip  DiagnosticForOutOfRangeInput=Warning  InternalRulePriority=Speed
      settings: InputPortMap=u0,u1,u2,u3,u4,u5
  Vflight Prelookup : PreLookup  BreakpointsData=LD.Propulsion.motor2.Vflight  ExtrapMethod=Linear
  Voltage Prelookup : PreLookup  BreakpointsData=LD.Propulsion.motor2.Voltage  ExtrapMethod=Linear
  Thrust : Outport
  Power : Outport  Port=2
  Current : Outport  Port=3
  RPM : Outport  Port=4
  wires:
  Height/1 -> Height Prelookup/1
  Vflight/1 -> Vflight Prelookup/1
  RPM Interpolation Using Prelookup/1 -> RPM/1  "RPM"
  Power Interpolation Using Prelookup/1 -> Power/1  "Power"
  Thrust Interpolation Using Prelookup/1 -> Thrust/1  "Thrust"
  Current Interpolation Using Prelookup/1 -> Current/1  "Current"
  Voltage/1 -> Voltage Prelookup/1
  Voltage Prelookup/1 -> [k1]
  Voltage Prelookup/2 -> [f1]
  Height Prelookup/1 -> [k2]
  Height Prelookup/2 -> [f2]
  Vflight Prelookup/2 -> [f3]
  Vflight Prelookup/1 -> [k3]
  [k1] -> Thrust Interpolation Using Prelookup/1
  [k1] -> Power Interpolation Using Prelookup/1
  [k1] -> Current Interpolation Using Prelookup/1
  [k1] -> RPM Interpolation Using Prelookup/1
  [f1] -> Thrust Interpolation Using Prelookup/2
  [k2] -> Thrust Interpolation Using Prelookup/3
  [k2] -> Power Interpolation Using Prelookup/3
  [k2] -> Current Interpolation Using Prelookup/3
  [k2] -> RPM Interpolation Using Prelookup/3
  [k3] -> Thrust Interpolation Using Prelookup/5
  [k3] -> Power Interpolation Using Prelookup/5
  [k3] -> Current Interpolation Using Prelookup/5
  [k3] -> RPM Interpolation Using Prelookup/5
  [f1] -> Power Interpolation Using Prelookup/2
  [f1] -> Current Interpolation Using Prelookup/2
  [f1] -> RPM Interpolation Using Prelookup/2
  [f2] -> RPM Interpolation Using Prelookup/4
  [f2] -> Current Interpolation Using Prelookup/4
  [f2] -> Power Interpolation Using Prelookup/4
  [f2] -> Thrust Interpolation Using Prelookup/4
  [f3] -> RPM Interpolation Using Prelookup/6
  [f3] -> Current Interpolation Using Prelookup/6
  [f3] -> Power Interpolation Using Prelookup/6
  [f3] -> Thrust Interpolation Using Prelookup/6

== system mainV02_3/LIBIS Plant/Propulsion/Motor_3/ESC_3 ==
  V_battery : Inport  Unit=V
  Throttle : Inport  Port=2  Unit=1
  Product : Product
  Product1 : Product
  eta_ESC : Constant  Value=LD.Propulsion.ESC3.eta
  isActive : Subsystem  Commented=on
  V_ESC : Outport  Unit=V
  wires:
  eta_ESC/1 -> Product/2
  V_battery/1 -> Product/1
  Product/1 -> Product1/1
  Product1/1 -> V_ESC/1
  Throttle/1 -> Product1/2
